simulink model "DRDistrictSystem"  (R2026a)
settings: Solver=FixedStepAuto  StopTime=200  FixedStep=1
settings Model: Creator=sudarshankumar  LastModifiedBy=sudarshankumar

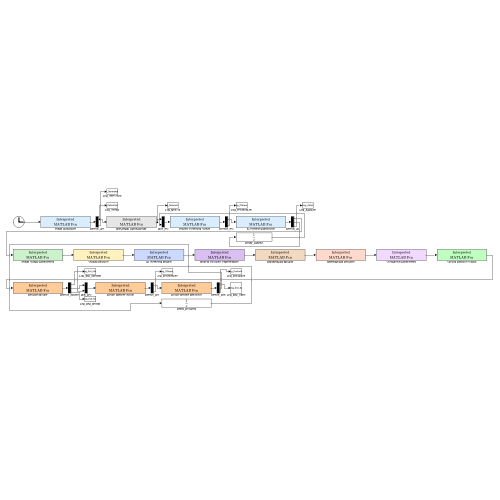
[thumbnail: Simulink's stored preview of the top-level diagram]
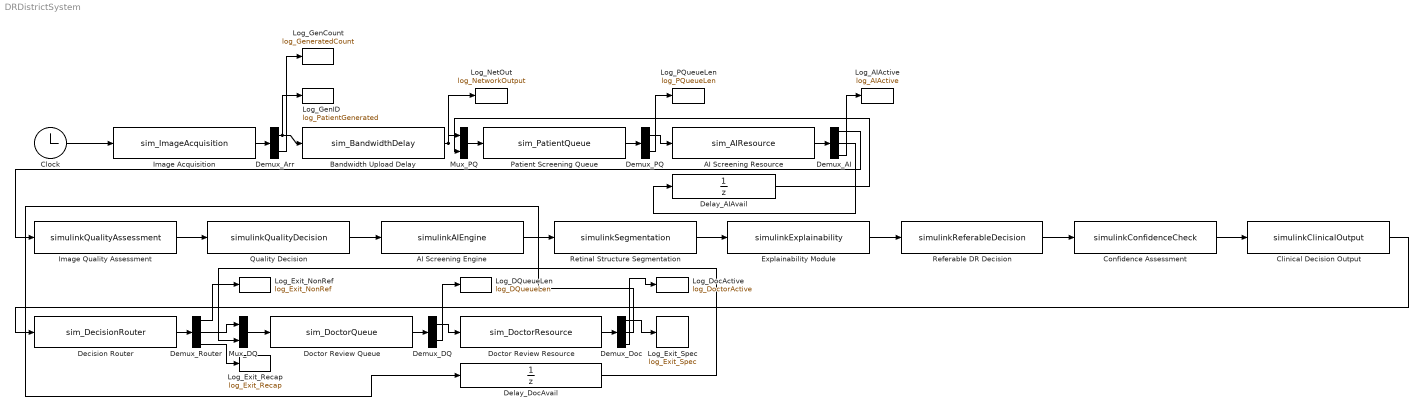
== system DRDistrictSystem ==
  AI Screening Engine : MATLABFcn  MATLABFcn=simulinkAIEngine  OutputDimensions=32
  AI Screening Resource : MATLABFcn  MATLABFcn=sim_AIResource  OutputDimensions=18
  Bandwidth Upload Delay : MATLABFcn  MATLABFcn=sim_BandwidthDelay  OutputDimensions=1
  Clinical Decision Output : MATLABFcn  MATLABFcn=simulinkClinicalOutput  OutputDimensions=32
  Clock : Clock
  Confidence Assessment : MATLABFcn  MATLABFcn=simulinkConfidenceCheck  OutputDimensions=32
  Decision Router : MATLABFcn  MATLABFcn=sim_DecisionRouter  OutputDimensions=64
  Delay_AIAvail : UnitDelay
  Delay_DocAvail : UnitDelay
  Demux_AI : Demux  Outputs="[16   1   1]"
  Demux_Arr : Demux  Outputs=2
  Demux_DQ : Demux  Outputs="[32   1]"
  Demux_Doc : Demux  Outputs="[32   1   1]"
  Demux_PQ : Demux  Outputs="[16   1]"
  Demux_Router : Demux  Outputs="[16  32  16]"
  Doctor Review Queue : MATLABFcn  MATLABFcn=sim_DoctorQueue  OutputDimensions=33
  Doctor Review Resource : MATLABFcn  MATLABFcn=sim_DoctorResource  OutputDimensions=34
  Explainability Module : MATLABFcn  MATLABFcn=simulinkExplainability  OutputDimensions=32
  Image Acquisition : MATLABFcn  MATLABFcn=sim_ImageAcquisition  OutputDimensions=2
  Image Quality Assessment : MATLABFcn  MATLABFcn=simulinkQualityAssessment  OutputDimensions=32
  Log_AIActive : ToWorkspace  VariableName=log_AIActive  SampleTime=-1
  Log_DQueueLen : ToWorkspace  VariableName=log_DQueueLen  SampleTime=-1
  Log_DocActive : ToWorkspace  VariableName=log_DoctorActive  SampleTime=-1
  Log_Exit_NonRef : ToWorkspace  VariableName=log_Exit_NonRef  SampleTime=-1
  Log_Exit_Recap : ToWorkspace  VariableName=log_Exit_Recap  SampleTime=-1
  Log_Exit_Spec : ToWorkspace  VariableName=log_Exit_Spec  SampleTime=-1
  Log_GenCount : ToWorkspace  VariableName=log_GeneratedCount  SampleTime=-1
  Log_GenID : ToWorkspace  VariableName=log_PatientGenerated  SampleTime=-1
  Log_NetOut : ToWorkspace  VariableName=log_NetworkOutput  SampleTime=-1
  Log_PQueueLen : ToWorkspace  VariableName=log_PQueueLen  SampleTime=-1
  Mux_DQ : Mux  Inputs=2
  Mux_PQ : Mux  Inputs=2
  Patient Screening Queue : MATLABFcn  MATLABFcn=sim_PatientQueue  OutputDimensions=17
  Quality Decision : MATLABFcn  MATLABFcn=simulinkQualityDecision  OutputDimensions=32
  Referable DR Decision : MATLABFcn  MATLABFcn=simulinkReferableDecision  OutputDimensions=32
  Retinal Structure Segmentation : MATLABFcn  MATLABFcn=simulinkSegmentation  OutputDimensions=32
  wires:
  Clock/1 -> Image Acquisition/1
  Image Acquisition/1 -> Demux_Arr/1
  Demux_Arr/1 -> Bandwidth Upload Delay/1, Log_GenID/1
  Demux_Arr/2 -> Log_GenCount/1
  Bandwidth Upload Delay/1 -> Mux_PQ/1, Log_NetOut/1
  Delay_AIAvail/1 -> Mux_PQ/2
  Mux_PQ/1 -> Patient Screening Queue/1
  Patient Screening Queue/1 -> Demux_PQ/1
  Demux_PQ/1 -> AI Screening Resource/1
  Demux_PQ/2 -> Log_PQueueLen/1
  AI Screening Resource/1 -> Demux_AI/1
  Demux_AI/1 -> Image Quality Assessment/1
  Demux_AI/2 -> Delay_AIAvail/1
  Demux_AI/3 -> Log_AIActive/1
  Image Quality Assessment/1 -> Quality Decision/1
  Quality Decision/1 -> AI Screening Engine/1
  AI Screening Engine/1 -> Retinal Structure Segmentation/1
  Retinal Structure Segmentation/1 -> Explainability Module/1
  Explainability Module/1 -> Referable DR Decision/1
  Referable DR Decision/1 -> Confidence Assessment/1
  Confidence Assessment/1 -> Clinical Decision Output/1
  Clinical Decision Output/1 -> Decision Router/1
  Decision Router/1 -> Demux_Router/1
  Demux_Router/1 -> Log_Exit_NonRef/1
  Demux_Router/3 -> Log_Exit_Recap/1
  Demux_Router/2 -> Mux_DQ/1
  Delay_DocAvail/1 -> Mux_DQ/2
  Mux_DQ/1 -> Doctor Review Queue/1
  Doctor Review Queue/1 -> Demux_DQ/1
  Demux_DQ/1 -> Doctor Review Resource/1
  Demux_DQ/2 -> Log_DQueueLen/1
  Doctor Review Resource/1 -> Demux_Doc/1
  Demux_Doc/1 -> Log_Exit_Spec/1
  Demux_Doc/2 -> Delay_DocAvail/1
  Demux_Doc/3 -> Log_DocActive/1
